simulink model "Aceleration and Thrust to attitude"  (R2023b)
settings: Solver=VariableStepAuto  StartTime=0.0  StopTime=10.0  RelTol=1e-3
undefined symbols (not defined in the file): g
libraries: vrlib x4, simulink x2, sharedutil x2
settings Model: Creator=Saif Mohamed  LastModifiedBy=saifg

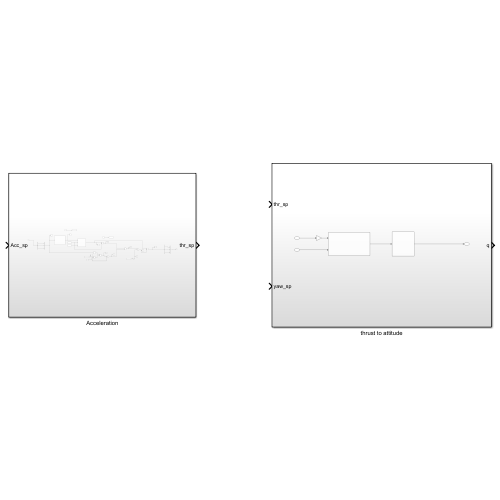
[thumbnail: Simulink's stored preview of the top-level diagram]
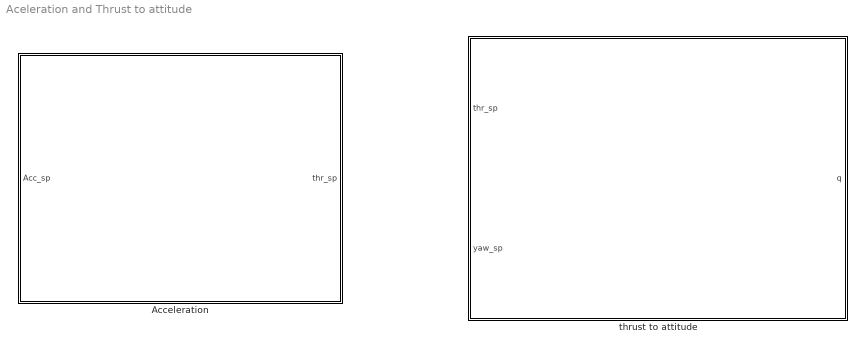
== system Aceleration and Thrust to attitude ==
  Acceleration : Subsystem
  thrust to attitude : Subsystem

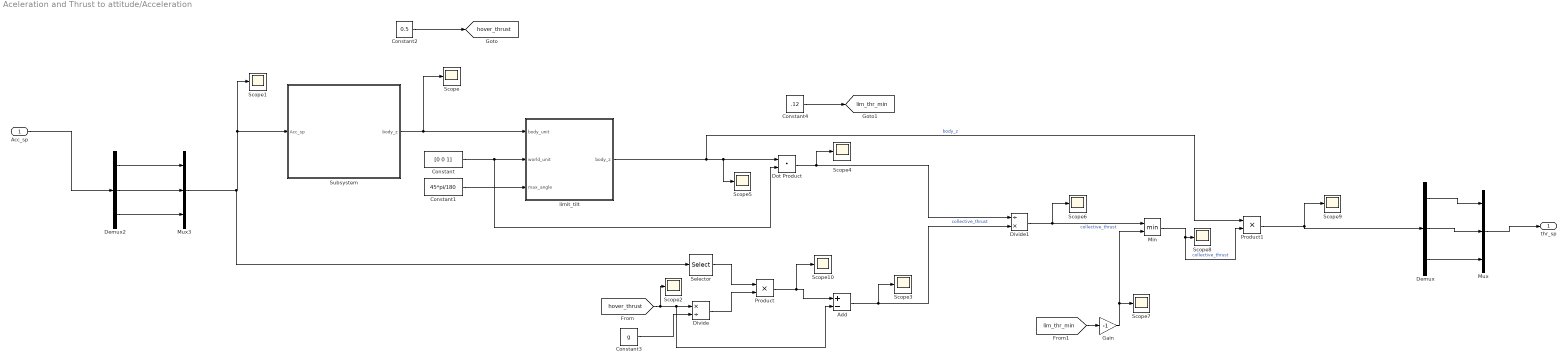
== system Aceleration and Thrust to attitude/Acceleration ==
  Acc_sp : Inport
  Add : Sum  Inputs=+-
  Constant : Constant  Value=[0 0 1]
  Constant1 : Constant  Value=45*pi/180
  Constant2 : Constant  Value=0.5
  Constant3 : Constant  Value=g
  Constant4 : Constant  Value=.12
  Demux : Demux  Outputs=3
  Demux2 : Demux  Outputs=3
  Divide : Product  Inputs=*/
  Divide1 : Product  Inputs=/*
  Dot Product : DotProduct  OutDataTypeStr=Inherit: Inherit via internal rule
  Gain : Gain  Gain=-1
  Min : MinMax  Inputs=2
  Mux : Mux  Inputs=3
  Mux3 : Mux  Inputs=3
  Product : Product
  Product1 : Product
  Scope{,1..10} (11 alike) : Scope
  Selector : Selector  InputPortWidth=3  IndexOptions=Index vector (dialog)  Indices=[3]  OutputSizes=1
  Subsystem : Subsystem
  limit_tilt : Subsystem
  thr_sp : Outport
  tag scope: hover_thrust=global, lim_thr_min=global
  wires:
  Subsystem/1(body_z) -> Scope/1, limit_tilt/1(body_unit)
  Constant/1 -> limit_tilt/2(world_unit), Dot Product/2
  Constant1/1 -> limit_tilt/3(max_angle)
  Constant2/1 -> [hover_thrust]
  [hover_thrust] -> Scope2/1, Add/2, Divide/1
  Constant3/1 -> Divide/2
  Selector/1 -> Product/1
  Divide/1 -> Product/2
  Product/1 -> Scope10/1, Add/1
  Add/1 -> Scope3/1, Divide1/2  "collective_thrust"
  limit_tilt/1(body_z) -> Product1/1, Scope5/1, Dot Product/1  "body_z"
  Dot Product/1 -> Scope4/1, Divide1/1
  Divide1/1 -> Min/1, Scope6/1  "collective_thrust"
  Constant4/1 -> [lim_thr_min]
  [lim_thr_min] -> Gain/1
  Gain/1 -> Min/2, Scope7/1
  Min/1 -> Scope8/1, Product1/2  "collective_thrust"
  Product1/1 -> Scope9/1, Demux/1
  Demux2/1 -> Mux3/1
  Demux2/2 -> Mux3/2
  Acc_sp/1 -> Demux2/1
  Mux3/1 -> Selector/1, Scope1/1, Subsystem/1(Acc_sp)
  Demux2/3 -> Mux3/3
  Demux/2 -> Mux/2
  Demux/1 -> Mux/1
  Demux/3 -> Mux/3
  Mux/1 -> thr_sp/1

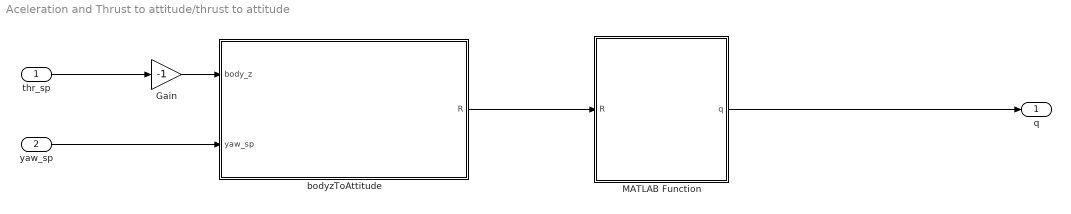
== system Aceleration and Thrust to attitude/thrust to attitude ==
  thr_sp : Inport
  yaw_sp : Inport  Port=2
  Gain : Gain  Gain=-1
  MATLAB Function : MATLAB Function  TreatAsAtomicUnit=on
  bodyzToAttitude : Subsystem
  q : Outport
  wires:
  thr_sp/1 -> Gain/1
  yaw_sp/1 -> bodyzToAttitude/2(yaw_sp)
  Gain/1 -> bodyzToAttitude/1(body_z)
  bodyzToAttitude/1(R) -> MATLAB Function/1(R)
  MATLAB Function/1(q) -> q/1

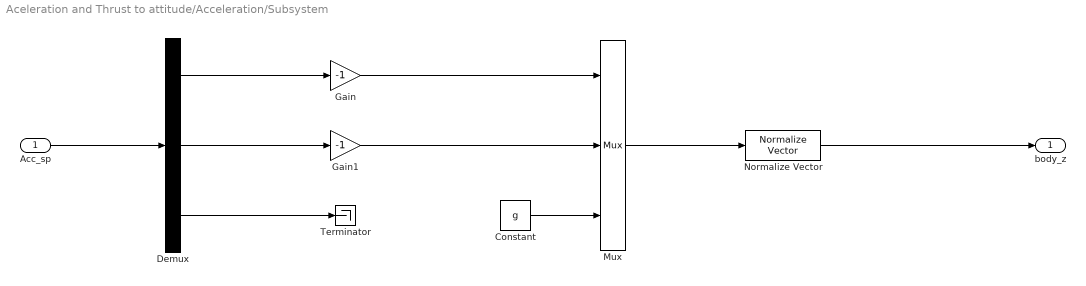
== system Aceleration and Thrust to attitude/Acceleration/Subsystem ==
  Acc_sp : Inport
  Constant : Constant  Value=g
  Demux : Demux  Outputs=3
  Gain : Gain  Gain=-1
  Gain1 : Gain  Gain=-1
  Mux : Mux  Inputs=3
  Normalize Vector : vrlib/Utilities/Normalize Vector  maxzero=0
  Terminator : Terminator
  body_z : Outport
  wires:
  Acc_sp/1 -> Demux/1
  Demux/1 -> Gain/1
  Demux/2 -> Gain1/1
  Demux/3 -> Terminator/1
  Gain1/1 -> Mux/2
  Gain/1 -> Mux/1
  Constant/1 -> Mux/3
  Mux/1 -> Normalize Vector/1
  Normalize Vector/1 -> body_z/1

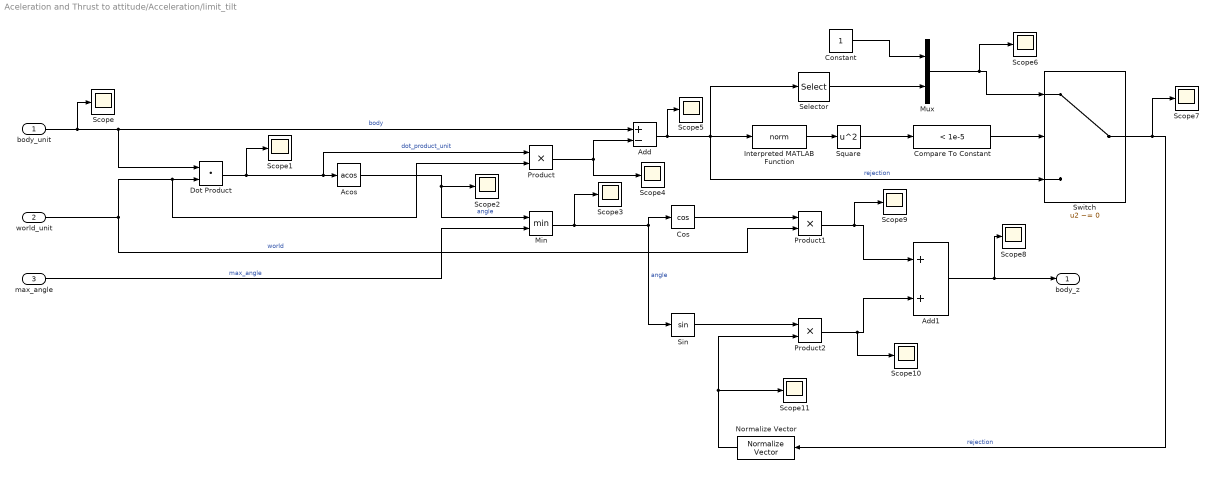
== system Aceleration and Thrust to attitude/Acceleration/limit_tilt ==
  body_unit : Inport
  world_unit : Inport  Port=2
  max_angle : Inport  Port=3
  Acos : Trigonometry  Operator=acos
  Add : Sum  Inputs=+-
  Add1 : Sum
  Compare To Constant : simulink/Logic and Bit Operations/Compare To Constant  relop=<  const=1e-5  OutDataTypeStr=boolean
  Constant : Constant
  Cos : Trigonometry  Operator=cos
  Dot Product : DotProduct  OutDataTypeStr=Inherit: Inherit via internal rule
  Interpreted MATLAB Function : MATLABFcn  MATLABFcn=norm
  Min : MinMax  Inputs=2
  Mux : Mux  Inputs=2
  Normalize Vector : vrlib/Utilities/Normalize Vector  maxzero=0
  Product : Product
  Product1 : Product
  Product2 : Product
  Scope{,1..11} (12 alike) : Scope
  Selector : Selector  InputPortWidth=3  IndexOptions=Index vector (dialog)  Indices=[2 3]  OutputSizes=1
  Sin : Trigonometry
  Square : Math  Operator=square
  Switch : Switch  Criteria=u2 ~= 0  SaturateOnIntegerOverflow=off  InputSameDT=off
  body_z : Outport
  wires:
  world_unit/1 -> Product/2, Dot Product/2, Product1/2  "world"
  body_unit/1 -> Scope/1, Add/1, Dot Product/1  "body"
  Dot Product/1 -> Scope1/1, Product/1, Acos/1  "dot_product_unit"
  Acos/1 -> Scope2/1, Min/1  "angle"
  max_angle/1 -> Min/2  "max_angle"
  Product/1 -> Scope4/1, Add/2
  Add/1 -> Scope5/1, Switch/3, Selector/1, Interpreted MATLAB Function/1  "rejection"
  Interpreted MATLAB Function/1 -> Square/1
  Square/1 -> Compare To Constant/1
  Compare To Constant/1 -> Switch/2
  Constant/1 -> Mux/1
  Mux/1 -> Scope6/1, Switch/1
  Selector/1 -> Mux/2
  Min/1 -> Scope3/1, Sin/1, Cos/1  "angle"
  Switch/1 -> Normalize Vector/1, Scope7/1  "rejection"
  Cos/1 -> Product1/1
  Sin/1 -> Product2/1
  Normalize Vector/1 -> Scope11/1, Product2/2
  Product2/1 -> Scope10/1, Add1/2
  Product1/1 -> Scope9/1, Add1/1
  Add1/1 -> Scope8/1, body_z/1

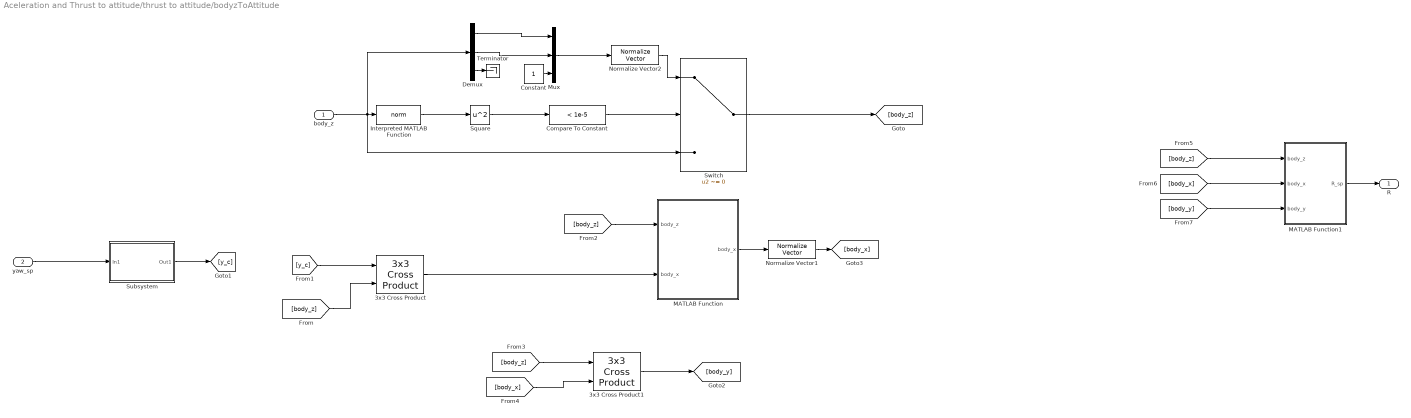
== system Aceleration and Thrust to attitude/thrust to attitude/bodyzToAttitude ==
  body_z : Inport
  yaw_sp : Inport  Port=2
  3x3 Cross Product : sharedutil/3x3 Cross Product  aMode=aMode
      settings: LibrarySourceBlock=aerolibutil/3x3 Cross Product
  3x3 Cross Product1 : sharedutil/3x3 Cross Product  aMode=aMode
      settings: LibrarySourceBlock=aerolibutil/3x3 Cross Product
  Compare To Constant : simulink/Logic and Bit Operations/Compare To Constant  relop=<  const=1e-5  OutDataTypeStr=boolean
  Constant : Constant
  Demux : Demux  Outputs=3
  Interpreted MATLAB Function : MATLABFcn  MATLABFcn=norm
  MATLAB Function : MATLAB Function  TreatAsAtomicUnit=on
  MATLAB Function1 : MATLAB Function  TreatAsAtomicUnit=on
  Mux : Mux  Inputs=3
  Normalize Vector1 : vrlib/Utilities/Normalize Vector  maxzero=0
  Normalize Vector2 : vrlib/Utilities/Normalize Vector  maxzero=0
  Square : Math  Operator=square
  Subsystem : Subsystem
  Switch : Switch  Criteria=u2 ~= 0  SaturateOnIntegerOverflow=off  InputSameDT=off
  Terminator : Terminator
  R : Outport
  wires:
  Interpreted MATLAB Function/1 -> Square/1
  Square/1 -> Compare To Constant/1
  Compare To Constant/1 -> Switch/2
  Demux/1 -> Mux/1
  Demux/2 -> Mux/2
  Constant/1 -> Mux/3
  Mux/1 -> Normalize Vector2/1
  Switch/1 -> [body_z]
  yaw_sp/1 -> Subsystem/1(In1)
  Subsystem/1(Out1) -> [y_c]
  [y_c] -> 3x3 Cross Product/1
  [body_z] -> 3x3 Cross Product/2
  [body_z] -> MATLAB Function/1(body_z)
  3x3 Cross Product/1 -> MATLAB Function/2("body_x ")
  MATLAB Function/1(body_x) -> Normalize Vector1/1
  Normalize Vector1/1 -> [body_x]
  [body_z] -> 3x3 Cross Product1/1
  [body_x] -> 3x3 Cross Product1/2
  3x3 Cross Product1/1 -> [body_y]
  [body_z] -> MATLAB Function1/1(body_z)
  [body_x] -> MATLAB Function1/2(body_x)
  [body_y] -> MATLAB Function1/3(body_y)
  MATLAB Function1/1(R_sp) -> R/1
  body_z/1 -> Switch/3, Demux/1, Interpreted MATLAB Function/1
  Demux/3 -> Terminator/1
  Normalize Vector2/1 -> Switch/1

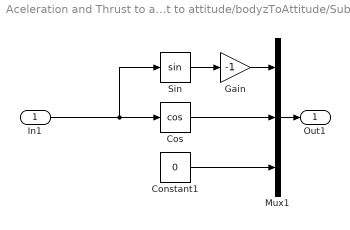
== system Aceleration and Thrust to attitude/thrust to attitude/bodyzToAttitude/Subsystem ==
  In1 : Inport
  Constant1 : Constant  Value=0
  Cos : Trigonometry  Operator=cos
  Gain : Gain  Gain=-1
  Mux1 : Mux  Inputs=3
  Sin : Trigonometry
  Out1 : Outport
  wires:
  In1/1 -> Sin/1, Cos/1
  Gain/1 -> Mux1/1
  Sin/1 -> Gain/1
  Constant1/1 -> Mux1/3
  Cos/1 -> Mux1/2
  Mux1/1 -> Out1/1

== matlab function Aceleration and Thrust to attitude/thrust to attitude/bodyzToAttitude/MATLAB Function1 ==
  data: body_z input; R_sp output; body_x input; body_y input
function R_sp = fcn(body_z,body_x,body_y)
R_sp=zeros(3,3);
for  i =1:3
		R_sp(i, 1) = body_x(i);
		R_sp(i, 2) = body_y(i);
		R_sp(i, 3) = body_z(i);
end

== matlab function Aceleration and Thrust to attitude/thrust to attitude/MATLAB Function ==
  data: R input; q output
function q = fcn(R)
    q = [0; 0; 0; 1];
    t = trace(R);
    if t > 0
        t = sqrt(1+t);
        q(1) = 0.5 * t;
        t = 0.5 / t;
        q(2) = (R(3,2) - R(2,3))*t;
        q(3) = (R(1,3) - R(3,1)) * t;
        q(4) = (R(2,1) - R(1,2)) * t;
    elseif R(1,1) > R(2,2) && R(1,1) > R(3,3)
        t = sqrt(1+R(1,1)-R(2,2)-R(3,3));
        q(2) = 0.5 * t;
        t = 0.5 / t;
        q(1) = (R(3,2) - R(2,3)) * t;
        q(3) = (R(2,1) + R(1,2)) * t;
        q(4) = (R(1,3) + R(3,1)) * t;
    elseif R(2,2) > R(3,3)
        t = sqrt(1 - R(1,1) + R(2,2) - R(3,3));
        q(3) = 0.5 * t;
        t = 0.5 / t;
        q(1) = (R(1,3) - R(3,1)) * t;
        q(2) = (R(2,1) + R(1,2)) * t;
        q(4) = (R(3,2) + R(2,3)) * t;
    else
        t = sqrt(1 - R(1,1) - R(2,2) + R(3,3));
        q(4) = 0.5 * t;
        t = 0.5 / t;
        q(1) = (R(2,1) - R(1,2)) * t;
        q(2) = (R(1,3) + R(3,1)) * t;
        q(3) = (R(3,2) + R(2,3)) * t;
    end
end

== matlab function Aceleration and Thrust to attitude/thrust to attitude/bodyzToAttitude/MATLAB Function ==
  data: body_z input; body_x output; body_x input
function body_x = fcn(body_z, body_x)

if (body_z(3)<0)
    body_x=-body_x;
end

if abs(body_z(3)) < 0.000001
    body_x(1)=0;
    body_x(2)=0;
    body_x(3)=1;

end
